simulink model "nmsRR"  (R2021a)
settings: Solver=ode15s  StartTime=0.0  StopTime=t  MaxStep=1e-2  RelTol=1e-2
StartFcn:
  | tic
StopFcn:
  | toc
  | 
  | 
  | %if GimbalLockFlag
  |  % fprintf(2, 'Almost reached Gimbal Lock of IMU. Simulation stopped.\n')
  | %end
  | 
  | %fprintf('Elapsed time: %4.2f sec (%4.2f%% realtime)\n', a, tout(end)/a*100)
undefined symbols (not defined in the file): Balance02, Balance13, BalanceTrunk, BasisStim, CompensateSwing, CompliantLeg, FlexAnkle, Ground, ICs, init_des_left, init_des_right, init_l_left, init_l_right, init_q_del, init_sensor_body, init_sensor_world, init_v_left, init_v_right, LateralControl, mParams, PreventKneeOverextension, StepDur, Target02, Target13, theta0, X, Y, Z
libraries: simulink_extras x133, nesl_utility x105, sm_lib x88, simulink x72, robotcorelib x5, dspinverses x5, dspswit3 x2, vrlib x2, robotmaniplib x1
(part 1 of 8)
settings Model: Creator=hgeyer  LastModifiedBy=reimajbi
settings SolverCC: ZeroCrossAlgorithm=Adaptive  AlgebraicLoopSolver=TrustRegion  MinimalZcImpactIntegration=on
settings OptimizationCC: EfficientMapNaN2IntZero=off
settings DebuggingCC: ReadBeforeWriteMsg=DisableAll  WriteAfterWriteMsg=DisableAll  WriteAfterReadMsg=DisableAll  IgnoredZcDiagnostic=none  MultiTaskDSMMsg=none  SFMachineParentedDataDiag=warning  ArithmeticOperatorsInVariantConditions=warning
settings HardwareCC: TargetBitPerLong=64  TargetBitPerPointer=64  TargetBitPerSizeT=64  TargetBitPerPtrDiffT=64  TargetLongLongMode=on  TargetIntDivRoundTo=Zero  TargetEndianess=LittleEndian  TargetWordSize=64  TargetHWDeviceType=MATLAB Host  ProdEqTarget=off
settings ModelReferenceCC: UpdateModelReferenceTargets=IfOutOfDate
settings SFSimCC: SFSimEcho=off  SimUseLocalCustomCode=off  CustomCodeUndefinedFunction=UseInterfaceOnly
settings CodeAppCC: MaxIdLength=128
settings SimscapeCC: SimscapeNormalizeSystem=off
settings ExplorerConfigSet: SimMechanicsOpenEditorOnUpdate=off  InternalSimMechanicsExplorerSettings="<ExplorerConfiguration><canonicalview>planar_xy</canonicalview><AnimationSetting><BasePlaybackSpeed>1.0</BasePlaybackSpeed><PlaybackSpeedFactor>1.0</PlaybackSpeedFactor></AnimationSetting><TilePanel><TileInfo><Tiles Columns=\"1\" Count=\"1\" Rows=\"1\"><Column Weight=\"1\"/><Row Weight=\"1\"/><Tile Height=\"1\" Width=\"1\" X=\"0\" Y=\"0\"/></Tiles></TileInfo><SceneInfo><SceneViewer><BGColor><R>0.60000002384185791</R><G>0.60000002384185791</G><B>0.60000002384185791</B></BGColor><Camera><DoPerspective>off</DoPerspective><Position><X>0.597774143722594631</X><Y>0.919449529340500282</Y><Z>14.1815791267909113</Z></Position><Center><X>0.597774143722594631</X><Y>0.919449529340500282</Y><Z>3.38181724401920292e-07</Z></Center><Up><X>0</X><Y>1</Y><Z>0</Z></Up><ViewLimDist>1</ViewLimDist><YLim>1.30566284997374105</YLim><XLim>1.60885047805753101</XLim></Camera></SceneViewer></SceneInfo></TilePanel><MechEditorPanel><Cameras/><GfxPanelCameraMap/><VideoCreator><PlaybackSpeedRatio>1.0</PlaybackSpeedRatio><FrameRate>30</FrameRate><VideoFormat>Motion JPEG AVI</VideoFormat><FrameSize>auto</FrameSize></VideoCreator></MechEditorPanel></ExplorerConfiguration>"

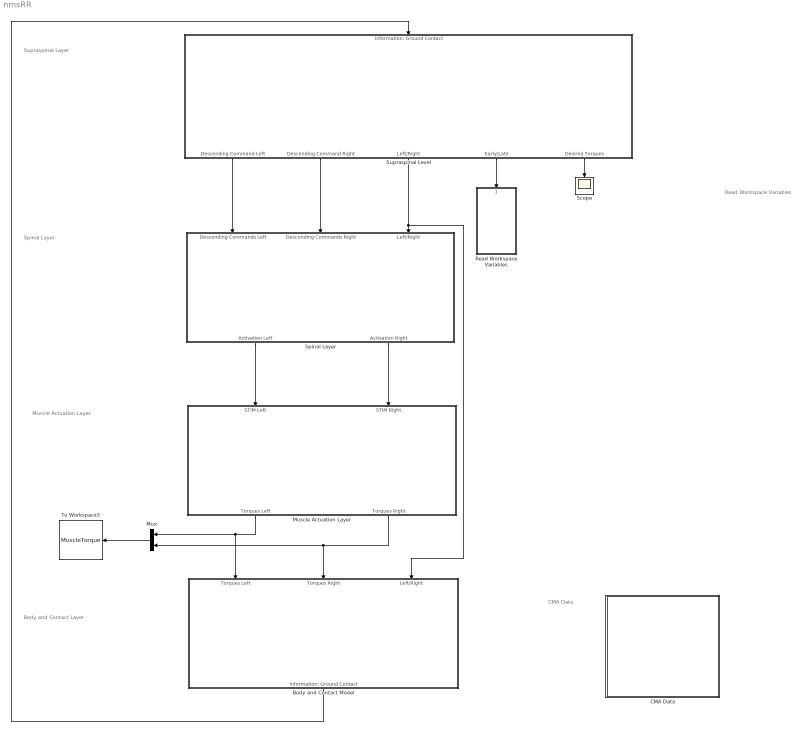
== system nmsRR ==
  note: Spinal Layer
  note: Muscle Actuation Layer
  note: Body and Contact Layer
  note: Supraspinal Layer
  note: CMA Data
  note: Read Workspace Variables
  Body and Contact Model : Subsystem
  CMA Data : Subsystem
  Muscle Actuation Layer : Subsystem
  Mux : Mux  Inputs=2
  Read Workspace Variables : Subsystem
  Scope : Scope
  Spinal Layer : Subsystem
  Supraspinal Level : Subsystem
  To Workspace3 : ToWorkspace  VariableName=MuscleTorque  SampleTime=-1
      settings: Save2DSignal=2-D array (concatenate along first dimension)
  wires:
  Spinal Layer/1(Activation Left) -> Muscle Actuation Layer/1(STIM Left)
  Spinal Layer/2(Activation Right) -> Muscle Actuation Layer/2(STIM Right)
  Muscle Actuation Layer/1(Torques Left) -> Mux/1, Body and Contact Model/1(Torques Left)
  Muscle Actuation Layer/2(Torques Right) -> Mux/2, Body and Contact Model/2(Torques Right)
  Supraspinal Level/1(Descending Command Left) -> Spinal Layer/1(Descending Commands Left)
  Supraspinal Level/2(Descending Command Right) -> Spinal Layer/2(Descending Commands Right)
  Supraspinal Level/3(Left/Right) -> Body and Contact Model/3(Left/Right), Spinal Layer/3(Left/Right)
  Supraspinal Level/4(Early/Late) -> Read Workspace Variables/1(Early/Late Swing)
  Body and Contact Model/1(Information: Ground Contact) -> Supraspinal Level/1(Information: Ground Contact)
  Mux/1 -> To Workspace3/1
  Supraspinal Level/5(Desired Torques) -> Scope/1

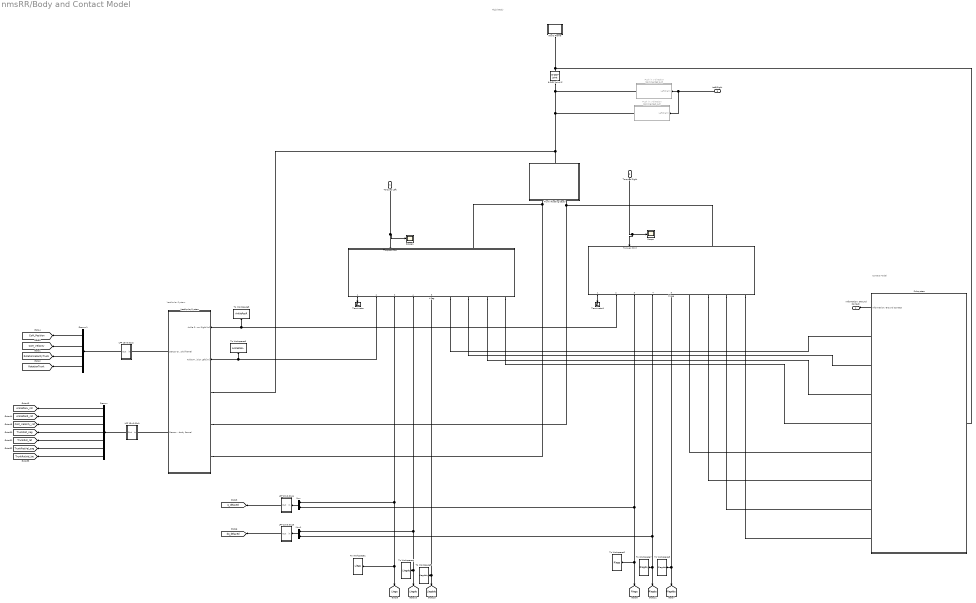
== system nmsRR/Body and Contact Model ==
  note: Rigid Body
  note: Contact Model
  note: Vestibular System
  Torques Left : Inport
  Torques Right : Inport  Port=2
  Left/Right : Inport  Port=3
  6-DOF Joint IC : sm_lib/Joints/6-DOF Joint  JointMode=Normal  SenseConstraintForce=off  SenseConstraintForceX=off  SenseConstraintForceY=off  SenseConstraintForceZ=off  SenseConstraintTorque=off  SenseConstraintTorqueX=off  SenseConstraintTorqueY=off  SenseConstraintTorqueZ=off  SenseTotalForce=off  SenseTotalForceX=off  SenseTotalForceY=off  SenseTotalForceZ=off  SenseTotalTorque=off  SenseTotalTorqueX=off  SenseTotalTorqueY=off  SenseTotalTorqueZ=off  CompositeWrenchDir=BaseOnFollower  CompositeWrenchFrame=FollowerFrame  PxEquilibriumPosition=0  PxEquilibriumPositionUnits=m  PxSpringStiffness=0  PxSpringStiffnessUnits=N/m  PxDampingCoefficient=0  PxDampingCoefficientUnits=N/(m/s)  PxTorqueActuationMode=NoTorque  PxMotionActuationMode=ComputedMotion  PxSensePosition=off  PxSenseVelocity=off  PxSenseAcceleration=off  PxSenseTorqueForce=off  PxSenseLowerLimitTorqueForce=off  PxSenseUpperLimitTorqueForce=off  PxLowerLimitSpecify=off  PxLowerLimitBound=-1  PxLowerLimitBoundUnits=m  PxLowerLimitStiffness=1e6  PxLowerLimitStiffnessUnits=N/m  PxLowerLimitDamping=1e3  PxLowerLimitDampingUnits=N/(m/s)  PxLowerLimitTransitionRegionWidth=1e-4  PxLowerLimitTransitionRegionWidthUnits=m  PxUpperLimitSpecify=off  PxUpperLimitBound=1  PxUpperLimitBoundUnits=m  PxUpperLimitStiffness=1e6  PxUpperLimitStiffnessUnits=N/m  PxUpperLimitDamping=1e3  PxUpperLimitDampingUnits=N/(m/s)  PxUpperLimitTransitionRegionWidth=1e-4  PxUpperLimitTransitionRegionWidthUnits=m  PxPositionTargetSpecify=on  PxPositionTargetPriority=High  PxPositionTargetValue=ICs.trunk.x0  PxPositionTargetValueUnits=m  PxVelocityTargetSpecify=on  PxVelocityTargetPriority=High  PxVelocityTargetValue=ICs.trunk.vx0  PxVelocityTargetValueUnits=m/s  PyEquilibriumPosition=0  PyEquilibriumPositionUnits=m  PySpringStiffness=0  PySpringStiffnessUnits=N/m  PyDampingCoefficient=0  PyDampingCoefficientUnits=N/(m/s)  PyTorqueActuationMode=NoTorque  PyMotionActuationMode=ComputedMotion  PySensePosition=off  PySenseVelocity=off  PySenseAcceleration=off  PySenseTorqueForce=off  PySenseLowerLimitTorqueForce=off  PySenseUpperLimitTorqueForce=off  PyLowerLimitSpecify=off  PyLowerLimitBound=-1  PyLowerLimitBoundUnits=m  PyLowerLimitStiffness=1e6  PyLowerLimitStiffnessUnits=N/m  PyLowerLimitDamping=1e3  PyLowerLimitDampingUnits=N/(m/s)  PyLowerLimitTransitionRegionWidth=1e-4  PyLowerLimitTransitionRegionWidthUnits=m  PyUpperLimitSpecify=off  PyUpperLimitBound=1  PyUpperLimitBoundUnits=m  PyUpperLimitStiffness=1e6  PyUpperLimitStiffnessUnits=N/m  PyUpperLimitDamping=1e3  PyUpperLimitDampingUnits=N/(m/s)  PyUpperLimitTransitionRegionWidth=1e-4  PyUpperLimitTransitionRegionWidthUnits=m  PyPositionTargetSpecify=on  PyPositionTargetPriority=High  PyPositionTargetValue=ICs.trunk.y0  PyPositionTargetValueUnits=m  PyVelocityTargetSpecify=off  PyVelocityTargetPriority=High  PyVelocityTargetValue=0  PyVelocityTargetValueUnits=m/s  PzEquilibriumPosition=0  PzEquilibriumPositionUnits=m  PzSpringStiffness=0  PzSpringStiffnessUnits=N/m  PzDampingCoefficient=0  PzDampingCoefficientUnits=N/(m/s)  PzTorqueActuationMode=NoTorque  PzMotionActuationMode=ComputedMotion  PzSensePosition=off  PzSenseVelocity=off  PzSenseAcceleration=off  PzSenseTorqueForce=off  PzSenseLowerLimitTorqueForce=off  PzSenseUpperLimitTorqueForce=off  PzLowerLimitSpecify=off  PzLowerLimitBound=-1  PzLowerLimitBoundUnits=m  PzLowerLimitStiffness=1e6  PzLowerLimitStiffnessUnits=N/m  PzLowerLimitDamping=1e3  PzLowerLimitDampingUnits=N/(m/s)  PzLowerLimitTransitionRegionWidth=1e-4  PzLowerLimitTransitionRegionWidthUnits=m  PzUpperLimitSpecify=off  PzUpperLimitBound=1  PzUpperLimitBoundUnits=m  PzUpperLimitStiffness=1e6  PzUpperLimitStiffnessUnits=N/m  PzUpperLimitDamping=1e3  PzUpperLimitDampingUnits=N/(m/s)  PzUpperLimitTransitionRegionWidth=1e-4  PzUpperLimitTransitionRegionWidthUnits=m  PzPositionTargetSpecify=on  PzPositionTargetPriority=High  PzPositionTargetValue=ICs.trunk.z0  PzPositionTargetValueUnits=m  PzVelocityTargetSpecify=on  PzVelocityTargetPriority=High  PzVelocityTargetValue=ICs.trunk.vz0  PzVelocityTargetValueUnits=m/s  SphDefPosRotationMethod=None  SphDefPosRotationAngleUnits=deg  SphDefPosRotationStandardAxis=+Z  SphDefPosRotationAngle=0.0  SphDefPosRotationArbitraryAxis=[0 0 1]  SphDefPosFollAlignAxisA=+X  SphDefPosBaseAlignAxisA=+Y  SphDefPosFollAlignAxisB=+Y  SphDefPosBaseAlignAxisB=+Z  SphDefPosRotationSequenceAxes=FollowerAxes  SphDefPosRotationSequence=XYX  SphDefPosRotationSequenceAngles=[0 0 0]  SphDefPosRotationSequenceAnglesUnits=deg  SphDefPosRotationMatrix=[1 0 0; 0 1 0; 0 0 1]  SphEqPosRotationMethod=None  SphEqPosRotationAngleUnits=deg  SphEqPosRotationStandardAxis=+Y  SphEqPosRotationAngle=0.0  SphEqPosRotationArbitraryAxis=[0 0 1]  SphEqPosFollAlignAxisA=+X  SphEqPosBaseAlignAxisA=+Y  SphEqPosFollAlignAxisB=+Y  SphEqPosBaseAlignAxisB=+Z  SphEqPosRotationSequenceAxes=FollowerAxes  SphEqPosRotationSequence=XYZ  SphEqPosRotationSequenceAngles=[0 0 -0.3]  SphEqPosRotationSequenceAnglesUnits=rad  SphEqPosRotationMatrix=[1 0 0; 0 1 0; 0 0 1]  SphSpringStiffness=0  SphSpringStiffnessUnits=N*m/deg  SphDampingCoefficient=0  SphDampingCoefficientUnits=N*m/(deg/s)  SphActuateTorqueX=off  SphActuateTorqueY=off  SphActuateTorqueZ=off  SphActuateTorque=on  SphTorqueActuationMode=NoTorque  SphMotionActuationMode=ComputedMotion  SphActuationFrame=BaseFrame  SphSensePosition=off  SphSenseVelocityX=off  SphSenseVelocityY=off  SphSenseVelocityZ=off  SphSenseVelocity=off  SphSenseAccelerationX=off  SphSenseAccelerationY=off  SphSenseAccelerationZ=off  SphSenseAcceleration=off  SphSenseTorqueX=off  SphSenseTorqueY=off  SphSenseTorqueZ=off  SphSenseTorqueForce=off  SphSenseLowerLimitTorqueMag=off  SphSenseUpperLimitTorqueMag=off  SphSensingFrame=BaseFrame  SphLowerLimitSpecify=off  SphLowerLimitBound=15  SphLowerLimitBoundUnits=deg  SphLowerLimitStiffness=1e4  SphLowerLimitStiffnessUnits=N*m/deg  SphLowerLimitDamping=10  SphLowerLimitDampingUnits=N*m/(deg/s)  SphLowerLimitTransitionRegionWidth=0.1  SphLowerLimitTransitionRegionWidthUnits=deg  SphUpperLimitSpecify=off  SphUpperLimitBound=45  SphUpperLimitBoundUnits=deg  SphUpperLimitStiffness=1e4  SphUpperLimitStiffnessUnits=N*m/deg  SphUpperLimitDamping=10  SphUpperLimitDampingUnits=N*m/(deg/s)  SphUpperLimitTransitionRegionWidth=0.1  SphUpperLimitTransitionRegionWidthUnits=deg  SphPositionTargetRotationMethod=RotationSequence  SphPositionTargetRotationAngleUnits=deg  SphPositionTargetRotationStandardAxis=+Z  SphPositionTargetRotationAngle=0.0  SphPositionTargetRotationArbitraryAxis=[0 0 1]  SphPositionTargetFollAlignAxisA=+X  SphPositionTargetBaseAlignAxisA=+Y  SphPositionTargetFollAlignAxisB=+Y  SphPositionTargetBaseAlignAxisB=+Z  SphPositionTargetRotationSequenceAxes=BaseAxes  SphPositionTargetRotationSequence=XZY  SphPositionTargetRotationSequenceAngles=[ICs.trunk.qR0 ICs.trunk.qP0 ICs.trunk.qY0 ]  SphPositionTargetRotationSequenceAnglesUnits=rad  SphPositionTargetRotationMatrix=[1 0 0; 0 1 0; 0 0 1]  SphPositionTargetSpecify=on  SphPositionTargetPriority=High  SphVelocityTargetValue=[ICs.trunk.qR0 ICs.trunk.qP0 ICs.trunk.qY0 ]  SphVelocityTargetValueUnits=deg/s  SphVelocityTargetSpecify=on  SphVelocityTargetPriority=High  SphVelocityTargetInFollowerFrame=on
  Demux : Demux  Outputs=7
  Demux1 : Demux
  L Leg : Subsystem
  LPF 13x0.01s1 : Subsystem
  LPF 13x0.01s2 : Subsystem
  LPF 13x0.01s3 : Subsystem
  LPF 13x0.01s4 : Subsystem
  Mux : Mux  Inputs=2
  Mux1 : Mux  Inputs=2
  Push in x-direction : Subsystem  Commented=on
  Push in y-direction : Subsystem  Commented=on
  R Leg : Subsystem
  Scope : Scope
  Scope1 : Scope
  Subsystem : Subsystem
  Terminator : Terminator
  Terminator1 : Terminator
  To Workspace1 : ToWorkspace  VariableName=Llegq  SampleTime=-1
      settings: Save2DSignal=2-D array (concatenate along first dimension)
  To Workspace2 : ToWorkspace  VariableName=Rlegq  SampleTime=-1
      settings: Save2DSignal=2-D array (concatenate along first dimension)
  To Workspace3 : ToWorkspace  VariableName=AnklePosR  SampleTime=-1
      settings: Save2DSignal=2-D array (concatenate along first dimension)
  To Workspace4 : ToWorkspace  VariableName=Llegdq  SampleTime=-1
      settings: Save2DSignal=2-D array (concatenate along first dimension)
  To Workspace5 : ToWorkspace  VariableName=Llegddq  SampleTime=-1
      settings: Save2DSignal=2-D array (concatenate along first dimension)
  To Workspace6 : ToWorkspace  VariableName=AnklePosL  SampleTime=-1
      settings: Save2DSignal=2-D array (concatenate along first dimension)
  To Workspace7 : ToWorkspace  VariableName=Rlegdq  SampleTime=-1
      settings: Save2DSignal=2-D array (concatenate along first dimension)
  To Workspace8 : ToWorkspace  VariableName=Rlegddq  SampleTime=-1
      settings: Save2DSignal=2-D array (concatenate along first dimension)
  Trunk (floating base) : Subsystem
  Vestibular System : Subsystem
  World Frame : Subsystem
  Information: Ground Contact : Outport
  tag scope: AnklePosL_rot=global, AnklePosR_rot=global, CoM_Position=global, CoM_Velocity=global, CoM_Velocity_rot=global, Llegddq=global, Llegdq=global, Llegq=global, Rlegddq=global, Rlegdq=global, Rlegq=global, RotationTrunk=global, RotationVelocityTrunk=global, TrunkRotVel_lat=global, TrunkRotVel_sag=global, TrunkRot_lat=global, TrunkRot_sag=global, dq_delayed=global, q_delayed=global
  wires:
  R Leg/4("Joint Velocities Right [rad/s] ") -> Mux1/2, To Workspace7/1, [Rlegdq]
  R Leg/5(Joint Accelerations Right [rad/s^2]) -> To Workspace8/1, [Rlegddq]
  R Leg/3(Joint Angles Right [rad]) -> Mux/2, To Workspace2/1, [Rlegq]
  L Leg/3(Joint Angles Left [rad]) -> Mux/1, To Workspace1/1, [Llegq]
  L Leg/5(Joint Accelerations Left [rad/s^2]) -> To Workspace5/1, [Llegddq]
  L Leg/4("Joint Velocities Left [rad/s] ") -> To Workspace4/1, [Llegdq], Mux1/1
  R Leg/2(Position Right Ankle [m]) -> To Workspace3/1, Vestibular System/1(Ankle Position Right [m])
  L Leg/2(" Position Left Ankle [m]") -> To Workspace6/1, Vestibular System/2(Ankle Position Left [m])
  Subsystem/1(Information: Ground Contact) -> Information: Ground Contact/1
  Demux1/2 -> [CoM_Velocity]
  Demux/3 -> [CoM_Velocity_rot]
  Vestibular System/2(Sensor Data (body frame)) -> LPF 13x0.01s1/1(in)
  Demux/5 -> [TrunkRot_lat]
  Demux/6 -> [TrunkRotVel_sag]
  Demux1/1 -> [CoM_Position]
  Demux/4 -> [TrunkRot_sag]
  Demux1/4 -> [RotationTrunk]
  Demux/2 -> [AnklePosR_rot]
  Demux1/3 -> [RotationVelocityTrunk]
  Demux/1 -> [AnklePosL_rot]
  Demux/7 -> [TrunkRotVel_lat]
  L Leg/1(Rotation Matrix Left Knee (world)) -> Terminator/1
  R Leg/1(Rotation Matrix Right Knee (World)) -> Terminator1/1
  Left/Right/1 -> Push in y-direction/1(Left/Right), Push in x-direction/1(Left/Right)
  Mux/1 -> LPF 13x0.01s4/1(in)
  Mux1/1 -> LPF 13x0.01s3/1(in)
  Torques Left/1 -> Scope1/1, L Leg/1(Torques [Nm])
  Torques Right/1 -> Scope/1, R Leg/1(Torques [Nm])
  LPF 13x0.01s2/1(Out) -> Demux1/1
  LPF 13x0.01s1/1(Out) -> Demux/1
  Vestibular System/1(Sensor Data (world frame)) -> LPF 13x0.01s2/1(in)
  LPF 13x0.01s4/1(Out) -> [q_delayed]
  LPF 13x0.01s3/1(Out) -> [dq_delayed]
  connections:
  Trunk (floating base)/RConn1 -- Vestibular System/LConn3 -- L Leg/LConn1
  World Frame/RConn1 -- Subsystem/LConn1 -- 6-DOF Joint IC/LConn1
  L Leg/RConn1 -- Subsystem/RConn1
  L Leg/RConn2 -- Subsystem/RConn2
  L Leg/RConn3 -- Subsystem/RConn3
  L Leg/RConn4 -- Subsystem/RConn4
  Subsystem/RConn5 -- R Leg/RConn1
  R Leg/RConn2 -- Subsystem/RConn6
  R Leg/RConn3 -- Subsystem/RConn7
  R Leg/RConn4 -- Subsystem/RConn8
  Vestibular System/LConn2 -- R Leg/LConn1 -- Trunk (floating base)/RConn2
  6-DOF Joint IC/RConn1 -- Push in x-direction/RConn1 -- Push in y-direction/RConn1 -- Vestibular System/LConn1 -- Trunk (floating base)/LConn1

== system nmsRR/CMA Data ==
  Mux : Mux  Inputs=7
  SS_dist1 : Subsystem  TreatAsAtomicUnit=on
  Step Counter : Subsystem
  check steady state : Subsystem
  wires:
  Step Counter/1(nStep) -> check steady state/2(nStep)
  [Contact_left] -> Step Counter/2(Step1), SS_dist1/Trigger
  [Contact_right] -> Step Counter/1(Step2)
  [Ball_right] -> Mux/1
  [AnklePosR] -> Mux/2
  [HipR] -> Mux/3
  [TRK_CG] -> Mux/4
  [HipL] -> Mux/5
  [Ball_left] -> Mux/6
  [AnklePosL] -> Mux/7
  Mux/1 -> check steady state/1(p)
  check steady state/1(SS_dist) -> SS_dist1/1(In1)

== system nmsRR/Muscle Actuation Layer ==
  note: Muscle Actuation Layer
  STIM Left : Inport
  STIM Right : Inport  Port=2
  Muscles Left : Subsystem
  Muscles Right : Subsystem
  Mux : Mux
  Mux1 : Mux
  Torques Left : Outport
  Torques Right : Outport  Port=2
  wires:
  STIM Left/1 -> Muscles Left/1(STIM Left)
  STIM Right/1 -> Muscles Right/1(STIM Right)
  Muscles Left/1(tauHipPitchL) -> Mux/1
  Muscles Left/2(tauHipRollL) -> Mux/2
  Muscles Left/3(tauKneeL) -> Mux/3
  Muscles Left/4(tauHipAnkleL) -> Mux/4
  Muscles Right/1(tauHipPitchR) -> Mux1/1
  Muscles Right/2(tauHipRollR) -> Mux1/2
  Muscles Right/3(tauKneeR) -> Mux1/3
  Muscles Right/4(tauHipAnkleR) -> Mux1/4
  Mux/1 -> Torques Left/1
  Mux1/1 -> Torques Right/1

== system nmsRR/Read Workspace Variables ==
  Early/Late Swing : Inport
  Constant : Constant  Value=0
  Constant1 : Constant  Value=CompliantLeg
  Constant10 : Constant  Value=theta0
  Constant12 : Constant  Value=BasisStim
  Constant15 : Constant  Value=LateralControl
  Constant2 : Constant  Value=CompensateSwing
  Constant3 : Constant  Value=Balance02
  Constant4 : Constant  Value=Target02
  Constant5 : Constant  Value=Balance13
  Constant6 : Constant  Value=Target13
  Constant7 : Constant  Value=PreventKneeOverextension
  Constant8 : Constant  Value=BalanceTrunk
  Constant9 : Constant  Value=FlexAnkle
  Demux : Demux
  Demux1 : Demux  Outputs=2
  Mux : Mux  Inputs=5
  Switch1 : Switch  Criteria=u2 > Threshold
  Switch2 : Switch  Criteria=u2 > Threshold
  tag scope: BasisStim=global, ControlParam=global, ControlParamLat=global, cd=global, cd_lat=global, cv=global, cv_lat=global, swh=global, swh_lat=global, swk=global, theta0=global
  wires:
  Constant2/1 -> Mux/5
  Constant5/1 -> Switch2/3
  Constant1/1 -> Mux/1
  Demux/2 -> [cv]
  Switch2/1 -> Demux/1
  Constant3/1 -> Switch2/1
  Mux/1 -> [ControlParam]
  Constant8/1 -> Mux/3
  Demux/3 -> [cd_lat]
  Constant9/1 -> Mux/4
  Constant15/1 -> [ControlParamLat]
  Demux/1 -> [cd]
  Constant12/1 -> [BasisStim]
  Constant7/1 -> Mux/2
  Demux/4 -> [cv_lat]
  Constant/1 -> [swh_lat]
  Early/Late Swing/1 -> Switch1/2, Switch2/2
  Constant6/1 -> Switch1/3
  Switch1/1 -> Demux1/1
  Constant4/1 -> Switch1/1
  Demux1/1 -> [swh]
  Demux1/2 -> [swk]
  Constant10/1 -> [theta0]

== system nmsRR/Spinal Layer ==
  Descending Commands Left : Inport
  Descending Commands Right : Inport  Port=2
  Left/Right : Inport  Port=3
  Stance Leg Control Left : Subsystem
  Stance Leg Control Right : Subsystem
  Stretch Reflex for Swing Leg Control : Subsystem
  Switch : Switch  Criteria=u2 > Threshold
  Switch1 : Switch  Criteria=u2 > Threshold
  Activation Left : Outport
  Activation Right : Outport  Port=2
  wires:
  Descending Commands Right/1 -> Stretch Reflex for Swing Leg Control/2(Descending Commands Right)
  Descending Commands Left/1 -> Stretch Reflex for Swing Leg Control/1(Descending Commands Left)
  Stance Leg Control Right/1(Activation Right) -> Switch/3
  Left/Right/1 -> Switch1/2, Switch/2
  Stretch Reflex for Swing Leg Control/1(Activation Left) -> Stance Leg Control Right/1(Activation Swing Left), Switch1/3
  Stance Leg Control Left/1(Activation Left) -> Switch1/1
  Stretch Reflex for Swing Leg Control/2(Activation Right) -> Stance Leg Control Left/1(Activation Swing Right), Switch/1
  Switch1/1 -> Activation Left/1
  Switch/1 -> Activation Right/1

== system nmsRR/Supraspinal Level ==
  note: Finite State Machine
  note: Descending Commands for Swing Leg Control
  note: input: ground contact
  note: output: descending commands
  Information: Ground Contact : Inport
  Early/ Late : Logic  Operator=OR  AllPortsSameDT=off  OutDataTypeStr=boolean
  Finite State Machine : Subsystem
  Left/ Right : Logic  Operator=OR  AllPortsSameDT=off  OutDataTypeStr=boolean
  Subsystem : Subsystem
  To Workspace1 : ToWorkspace  VariableName=LateRight  SampleTime=-1
      settings: Save2DSignal=2-D array (concatenate along first dimension)
  To Workspace2 : ToWorkspace  VariableName=EarlyRight  SampleTime=-1
      settings: Save2DSignal=2-D array (concatenate along first dimension)
  To Workspace3 : ToWorkspace  VariableName=EarlyLeft  SampleTime=-1
      settings: Save2DSignal=2-D array (concatenate along first dimension)
  To Workspace4 : ToWorkspace  VariableName=Contact  SampleTime=-1
      settings: Save2DSignal=2-D array (concatenate along first dimension)
  To Workspace5 : ToWorkspace  VariableName=LateLeft  SampleTime=-1
      settings: Save2DSignal=2-D array (concatenate along first dimension)
  Descending Command Left : Outport
  Descending Command Right : Outport  Port=2
  Left/Right : Outport  Port=3
  Early/Late : Outport  Port=4
  Desired Torques : Outport  Port=5
  wires:
  Finite State Machine/3(Early Left Swing) -> Early/ Late/2, To Workspace3/1
  Left/ Right/1 -> Left/Right/1, Subsystem/2(Left/Right)
  Finite State Machine/1(Early Right Swing) -> To Workspace2/1, Left/ Right/1, Early/ Late/1
  Finite State Machine/4(Late Left Swing) -> To Workspace5/1
  Finite State Machine/2(Late Right Swing) -> Left/ Right/2, To Workspace1/1
  Early/ Late/1 -> Early/Late/1, Subsystem/1(Early/Late Swing)
  Information: Ground Contact/1 -> Finite State Machine/1(Information: Ground Contact), To Workspace4/1
  Subsystem/1(Descending Command Left) -> Descending Command Left/1
  Subsystem/2(Descending Command Right) -> Descending Command Right/1
  Subsystem/3(Desired Torques) -> Desired Torques/1

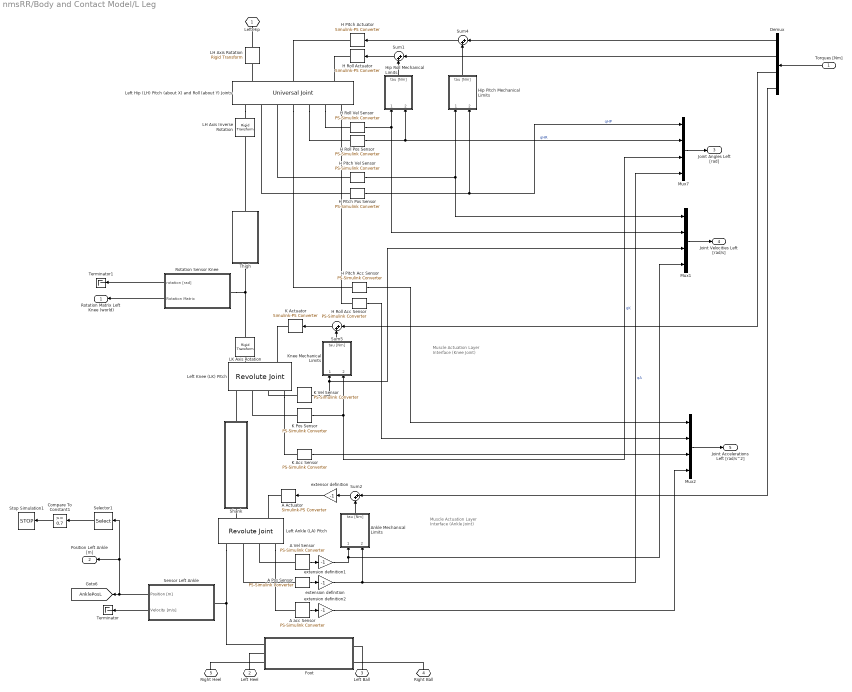
== system nmsRR/Body and Contact Model/L Leg ==
  note: Muscle Actuation
      | Layer Interface
      | (Ankle Joint)
  note: Muscle Actuation
      | Layer Interface
      | (Knee Joint)
  Torques [Nm] : Inport
  " K Actuator" : nesl_utility/Simulink-PS Converter  PhysicalDomain=network_engine_domain  SubClassName=ps_input  LeftPortType=input  RightPortType=output  PseudoPeriodic=off  Frequencies=[]  NoiseDistribution=none  NoiseParameters=[]  Unit=N*m  AffineConversion=off  FilteringAndDerivatives=zero  SimscapeFilterOrder=1  InputFilterTimeConstant=.001  UdotUserProvided=0
      settings: SourceProductBaseCode=PW,SS
  A Actuator : nesl_utility/Simulink-PS Converter  PhysicalDomain=network_engine_domain  SubClassName=ps_input  LeftPortType=input  RightPortType=output  PseudoPeriodic=off  Frequencies=[]  NoiseDistribution=none  NoiseParameters=[]  Unit=N*m  AffineConversion=off  FilteringAndDerivatives=zero  SimscapeFilterOrder=1  InputFilterTimeConstant=.001  UdotUserProvided=0
      settings: SourceProductBaseCode=PW,SS
  A Pos Sensor : nesl_utility/PS-Simulink Converter  PhysicalDomain=network_engine_domain  SubClassName=ps_output  LeftPortType=input  RightPortType=output  PseudoPeriodic=off  Frequencies=[]  Unit=rad  AffineConversion=off
      settings: SourceProductBaseCode=PW,SS
  A Vel Sensor : nesl_utility/PS-Simulink Converter  PhysicalDomain=network_engine_domain  SubClassName=ps_output  LeftPortType=input  RightPortType=output  PseudoPeriodic=off  Frequencies=[]  Unit=rad/s  AffineConversion=off
      settings: SourceProductBaseCode=PW,SS
  A acc Sensor : nesl_utility/PS-Simulink Converter  PhysicalDomain=network_engine_domain  SubClassName=ps_output  LeftPortType=input  RightPortType=output  PseudoPeriodic=off  Frequencies=[]  Unit=rad/(s^2)  AffineConversion=off
      settings: SourceProductBaseCode=PW,SS
  Ankle Mechanical Limits : Subsystem
  Compare To Constant1 : simulink/Logic and Bit Operations/Compare To Constant  relop=>=  const=0.7  OutDataTypeStr=boolean
  Demux : Demux
  Foot : Subsystem
  H Pitch Actuator : nesl_utility/Simulink-PS Converter  PhysicalDomain=network_engine_domain  SubClassName=ps_input  LeftPortType=input  RightPortType=output  PseudoPeriodic=off  Frequencies=[]  NoiseDistribution=none  NoiseParameters=[]  Unit=N*m  AffineConversion=off  FilteringAndDerivatives=zero  SimscapeFilterOrder=1  InputFilterTimeConstant=.001  UdotUserProvided=0
      settings: SourceProductBaseCode=PW,SS
  H Pitch Acc Sensor : nesl_utility/PS-Simulink Converter  PhysicalDomain=network_engine_domain  SubClassName=ps_output  LeftPortType=input  RightPortType=output  PseudoPeriodic=off  Frequencies=[]  Unit=rad/(s^2)  AffineConversion=off
      settings: SourceProductBaseCode=PW,SS
  H Pitch Pos Sensor : nesl_utility/PS-Simulink Converter  PhysicalDomain=network_engine_domain  SubClassName=ps_output  LeftPortType=input  RightPortType=output  PseudoPeriodic=off  Frequencies=[]  Unit=rad  AffineConversion=off
      settings: SourceProductBaseCode=PW,SS
  H Pitch Vel Sensor : nesl_utility/PS-Simulink Converter  PhysicalDomain=network_engine_domain  SubClassName=ps_output  LeftPortType=input  RightPortType=output  PseudoPeriodic=off  Frequencies=[]  Unit=rad/s  AffineConversion=off
      settings: SourceProductBaseCode=PW,SS
  H Roll Actuator : nesl_utility/Simulink-PS Converter  PhysicalDomain=network_engine_domain  SubClassName=ps_input  LeftPortType=input  RightPortType=output  PseudoPeriodic=off  Frequencies=[]  NoiseDistribution=none  NoiseParameters=[]  Unit=N*m  AffineConversion=off  FilteringAndDerivatives=zero  SimscapeFilterOrder=1  InputFilterTimeConstant=.001  UdotUserProvided=0
      settings: SourceProductBaseCode=PW,SS
  H Roll Acc Sensor : nesl_utility/PS-Simulink Converter  PhysicalDomain=network_engine_domain  SubClassName=ps_output  LeftPortType=input  RightPortType=output  PseudoPeriodic=off  Frequencies=[]  Unit=rad/(s^2)  AffineConversion=off
      settings: SourceProductBaseCode=PW,SS
  H Roll Pos Sensor : nesl_utility/PS-Simulink Converter  PhysicalDomain=network_engine_domain  SubClassName=ps_output  LeftPortType=input  RightPortType=output  PseudoPeriodic=off  Frequencies=[]  Unit=rad  AffineConversion=off
      settings: SourceProductBaseCode=PW,SS
  "H Roll Vel Sensor " : nesl_utility/PS-Simulink Converter  PhysicalDomain=network_engine_domain  SubClassName=ps_output  LeftPortType=input  RightPortType=output  PseudoPeriodic=off  Frequencies=[]  Unit=rad/s  AffineConversion=off
      settings: SourceProductBaseCode=PW,SS
  Hip Pitch Mechanical Limits : Subsystem
  Hip Roll Mechanical Limits : Subsystem
  K Acc Sensor : nesl_utility/PS-Simulink Converter  PhysicalDomain=network_engine_domain  SubClassName=ps_output  LeftPortType=input  RightPortType=output  PseudoPeriodic=off  Frequencies=[]  Unit=rad/(s^2)  AffineConversion=off
      settings: SourceProductBaseCode=PW,SS
  K Pos Sensor : nesl_utility/PS-Simulink Converter  PhysicalDomain=network_engine_domain  SubClassName=ps_output  LeftPortType=input  RightPortType=output  PseudoPeriodic=off  Frequencies=[]  Unit=rad  AffineConversion=off
      settings: SourceProductBaseCode=PW,SS
  K Vel Sensor : nesl_utility/PS-Simulink Converter  PhysicalDomain=network_engine_domain  SubClassName=ps_output  LeftPortType=input  RightPortType=output  PseudoPeriodic=off  Frequencies=[]  Unit=rad/s  AffineConversion=off
      settings: SourceProductBaseCode=PW,SS
  Knee Mechanical Limits : Subsystem
  LH Axis Inverse Rotation : sm_lib/Frames and Transforms/Rigid Transform  TranslationMethod=None  TranslationStandardOffset=-0.2  TranslationLengthUnit=m  TranslationStandardAxis=+Y  TranslationCartesianOffset=0  TranslationROffset=0  TranslationROffsetUnits=m  TranslationZOffset=0  TranslationZOffsetUnits=m  TranslationThetaOffset=0  TranslationThetaOffsetUnits=deg  RotationMethod=RotationSequence  RotationAngleUnits=deg  RotationStandardAxis=+X  RotationAngle=-90  RotationArbitraryAxis=[0 0 1]  FollAlignAxisA=+X  BaseAlignAxisA=+Y  FollAlignAxisB=+Y  BaseAlignAxisB=+Z  RotationSequenceAxes=BaseAxes  RotationSequence=YXY  RotationSequenceAngles=[-90 -90 0]  RotationSequenceAnglesUnits=deg  RotationMatrix=[1 0 0; 0 1 0; 0 0 1]
  LH Axis Rotation : sm_lib/Frames and Transforms/Rigid Transform  TranslationMethod=None  TranslationStandardOffset=-0.2  TranslationLengthUnit=m  TranslationStandardAxis=+Y  TranslationCartesianOffset=0  TranslationROffset=0  TranslationROffsetUnits=m  TranslationZOffset=0  TranslationZOffsetUnits=m  TranslationThetaOffset=0  TranslationThetaOffsetUnits=deg  RotationMethod=RotationSequence  RotationAngleUnits=deg  RotationStandardAxis=+X  RotationAngle=90  RotationArbitraryAxis=[0 0 1]  FollAlignAxisA=+X  BaseAlignAxisA=+Y  FollAlignAxisB=+Y  BaseAlignAxisB=+Z  RotationSequenceAxes=FollowerAxes  RotationSequence=XZX  RotationSequenceAngles=[-90 90 0]  RotationSequenceAnglesUnits=deg  RotationMatrix=[1 0 0; 0 1 0; 0 0 1]
  LK Axis Rotation : sm_lib/Frames and Transforms/Rigid Transform  TranslationMethod=None  TranslationStandardOffset=-0.5  TranslationLengthUnit=m  TranslationStandardAxis=+Y  TranslationCartesianOffset=0  TranslationROffset=0  TranslationROffsetUnits=m  TranslationZOffset=0  TranslationZOffsetUnits=m  TranslationThetaOffset=0  TranslationThetaOffsetUnits=deg  RotationMethod=RotationSequence  RotationAngleUnits=deg  RotationStandardAxis=+X  RotationAngle=-90  RotationArbitraryAxis=[0 0 1]  FollAlignAxisA=+X  BaseAlignAxisA=+Y  FollAlignAxisB=+Y  BaseAlignAxisB=+Z  RotationSequenceAxes=BaseAxes  RotationSequence=ZXZ  RotationSequenceAngles=[180 0 0]  RotationSequenceAnglesUnits=deg  RotationMatrix=[1 0 0; 0 1 0; 0 0 1]
  Left Ankle (LA) Pitch : sm_lib/Joints/Revolute Joint  JointMode=Normal  SenseConstraintForce=off  SenseConstraintForceX=off  SenseConstraintForceY=off  SenseConstraintForceZ=off  SenseConstraintTorque=off  SenseConstraintTorqueX=off  SenseConstraintTorqueY=off  SenseConstraintTorqueZ=off  SenseTotalForce=off  SenseTotalForceX=off  SenseTotalForceY=off  SenseTotalForceZ=off  SenseTotalTorque=off  SenseTotalTorqueX=off  SenseTotalTorqueY=off  SenseTotalTorqueZ=off  CompositeWrenchDir=FollowerOnBase  CompositeWrenchFrame=FollowerFrame  EquilibriumPosition=0  EquilibriumPositionUnits=deg  SpringStiffness=0  SpringStiffnessUnits=N*m/deg  DampingCoefficient=0  DampingCoefficientUnits=N*m/(deg/s)  TorqueActuationMode=InputTorque  MotionActuationMode=ComputedMotion  SensePosition=on  SenseVelocity=on  SenseAcceleration=on  SenseTorqueForce=off  SenseLowerLimitTorqueForce=off  SenseUpperLimitTorqueForce=off  LowerLimitSpecify=off  LowerLimitBound=-90  LowerLimitBoundUnits=deg  LowerLimitStiffness=1e4  LowerLimitStiffnessUnits=N*m/deg  LowerLimitDamping=10  LowerLimitDampingUnits=N*m/(deg/s)  LowerLimitTransitionRegionWidth=0.1  LowerLimitTransitionRegionWidthUnits=deg  UpperLimitSpecify=off  UpperLimitBound=90  UpperLimitBoundUnits=deg  UpperLimitStiffness=1e4  UpperLimitStiffnessUnits=N*m/deg  UpperLimitDamping=10  UpperLimitDampingUnits=N*m/(deg/s)  UpperLimitTransitionRegionWidth=0.1  UpperLimitTransitionRegionWidthUnits=deg  PositionTargetSpecify=on  PositionTargetPriority=High  PositionTargetValue=-ICs.lLeg.ankle.qP0  PositionTargetValueUnits=rad  VelocityTargetSpecify=on  VelocityTargetPriority=High  VelocityTargetValue=0  VelocityTargetValueUnits=rad/s
  Left Hip (LH) Pitch (about X) and Roll (about Y) Joints : sm_lib/Joints/Universal Joint  JointMode=Normal  SenseConstraintForce=off  SenseConstraintForceX=off  SenseConstraintForceY=off  SenseConstraintForceZ=off  SenseConstraintTorque=off  SenseConstraintTorqueX=off  SenseConstraintTorqueY=off  SenseConstraintTorqueZ=off  SenseTotalForce=off  SenseTotalForceX=off  SenseTotalForceY=off  SenseTotalForceZ=off  SenseTotalTorque=off  SenseTotalTorqueX=off  SenseTotalTorqueY=off  SenseTotalTorqueZ=off  CompositeWrenchDir=FollowerOnBase  CompositeWrenchFrame=FollowerFrame  RxEquilibriumPosition=0  RxEquilibriumPositionUnits=deg  RxSpringStiffness=0  RxSpringStiffnessUnits=N*m/deg  RxDampingCoefficient=0  RxDampingCoefficientUnits=N*m/(deg/s)  RxTorqueActuationMode=InputTorque  RxMotionActuationMode=ComputedMotion  RxSensePosition=on  RxSenseVelocity=on  RxSenseAcceleration=on  RxSenseTorqueForce=off  RxSenseLowerLimitTorqueForce=off  RxSenseUpperLimitTorqueForce=off  RxLowerLimitSpecify=off  RxLowerLimitBound=-90  RxLowerLimitBoundUnits=deg  RxLowerLimitStiffness=1e4  RxLowerLimitStiffnessUnits=N*m/deg  RxLowerLimitDamping=10  RxLowerLimitDampingUnits=N*m/(deg/s)  RxLowerLimitTransitionRegionWidth=0.1  RxLowerLimitTransitionRegionWidthUnits=deg  RxUpperLimitSpecify=off  RxUpperLimitBound=90  RxUpperLimitBoundUnits=deg  RxUpperLimitStiffness=1e4  RxUpperLimitStiffnessUnits=N*m/deg  RxUpperLimitDamping=10  RxUpperLimitDampingUnits=N*m/(deg/s)  RxUpperLimitTransitionRegionWidth=0.1  RxUpperLimitTransitionRegionWidthUnits=deg  RxPositionTargetSpecify=on  RxPositionTargetPriority=High  RxPositionTargetValue=ICs.lLeg.hip.qP0  RxPositionTargetValueUnits=rad  RxVelocityTargetSpecify=on  RxVelocityTargetPriority=High  RxVelocityTargetValue=0  RxVelocityTargetValueUnits=rad/s  RyEquilibriumPosition=0  RyEquilibriumPositionUnits=deg  RySpringStiffness=0  RySpringStiffnessUnits=N*m/deg  RyDampingCoefficient=0  RyDampingCoefficientUnits=N*m/(deg/s)  RyTorqueActuationMode=InputTorque  RyMotionActuationMode=ComputedMotion  RySensePosition=on  RySenseVelocity=on  RySenseAcceleration=on  RySenseTorqueForce=off  RySenseLowerLimitTorqueForce=off  RySenseUpperLimitTorqueForce=off  RyLowerLimitSpecify=off  RyLowerLimitBound=-90  RyLowerLimitBoundUnits=deg  RyLowerLimitStiffness=1e4  RyLowerLimitStiffnessUnits=N*m/deg  RyLowerLimitDamping=10  RyLowerLimitDampingUnits=N*m/(deg/s)  RyLowerLimitTransitionRegionWidth=0.1  RyLowerLimitTransitionRegionWidthUnits=deg  RyUpperLimitSpecify=off  RyUpperLimitBound=90  RyUpperLimitBoundUnits=deg  RyUpperLimitStiffness=1e4  RyUpperLimitStiffnessUnits=N*m/deg  RyUpperLimitDamping=10  RyUpperLimitDampingUnits=N*m/(deg/s)  RyUpperLimitTransitionRegionWidth=0.1  RyUpperLimitTransitionRegionWidthUnits=deg  RyPositionTargetSpecify=on  RyPositionTargetPriority=High  RyPositionTargetValue=ICs.lLeg.hip.qR0  RyPositionTargetValueUnits=rad  RyVelocityTargetSpecify=on  RyVelocityTargetPriority=High  RyVelocityTargetValue=0  RyVelocityTargetValueUnits=rad/s
  Left Knee (LK) Pitch : sm_lib/Joints/Revolute Joint  JointMode=Normal  SenseConstraintForce=off  SenseConstraintForceX=off  SenseConstraintForceY=off  SenseConstraintForceZ=off  SenseConstraintTorque=off  SenseConstraintTorqueX=off  SenseConstraintTorqueY=off  SenseConstraintTorqueZ=off  SenseTotalForce=off  SenseTotalForceX=off  SenseTotalForceY=off  SenseTotalForceZ=off  SenseTotalTorque=off  SenseTotalTorqueX=off  SenseTotalTorqueY=off  SenseTotalTorqueZ=off  CompositeWrenchDir=FollowerOnBase  CompositeWrenchFrame=FollowerFrame  EquilibriumPosition=0  EquilibriumPositionUnits=deg  SpringStiffness=0  SpringStiffnessUnits=N*m/deg  DampingCoefficient=0  DampingCoefficientUnits=N*m/(deg/s)  TorqueActuationMode=InputTorque  MotionActuationMode=ComputedMotion  SensePosition=on  SenseVelocity=on  SenseAcceleration=on  SenseTorqueForce=off  SenseLowerLimitTorqueForce=off  SenseUpperLimitTorqueForce=off  LowerLimitSpecify=off  LowerLimitBound=-90  LowerLimitBoundUnits=deg  LowerLimitStiffness=1e4  LowerLimitStiffnessUnits=N*m/deg  LowerLimitDamping=10  LowerLimitDampingUnits=N*m/(deg/s)  LowerLimitTransitionRegionWidth=0.1  LowerLimitTransitionRegionWidthUnits=deg  UpperLimitSpecify=off  UpperLimitBound=90  UpperLimitBoundUnits=deg  UpperLimitStiffness=1e4  UpperLimitStiffnessUnits=N*m/deg  UpperLimitDamping=10  UpperLimitDampingUnits=N*m/(deg/s)  UpperLimitTransitionRegionWidth=0.1  UpperLimitTransitionRegionWidthUnits=deg  PositionTargetSpecify=on  PositionTargetPriority=High  PositionTargetValue=ICs.lLeg.knee.qP0  PositionTargetValueUnits=rad  VelocityTargetSpecify=on  VelocityTargetPriority=High  VelocityTargetValue=0  VelocityTargetValueUnits=rad/s
  Mux1 : Mux
  Mux2 : Mux
  Mux7 : Mux
  Rotation Sensor Knee : Subsystem
  Selector1 : Selector  InputPortWidth=3  IndexOptions=Index vector (dialog)  Indices=[2]  OutputSizes=1
  Sensor Left Ankle : Subsystem
  Shank : Subsystem
  Stop Simulation1 : Stop
  Sum{1..2,4..5} (4 alike) : Sum  Inputs=|++
  Terminator : Terminator
  Terminator1 : Terminator
  Thigh : Subsystem
  extension definition : Gain  Gain=-1
  extension definition1 : Gain  Gain=-1
  extension definition2 : Gain  Gain=-1
  extensor definition : Gain  Gain=-1
  Left Hip : PMIOPort  Side=Left
  Left Heel : PMIOPort  Port=2  Side=Right
  Left Ball : PMIOPort  Port=3  Side=Right
  Right Ball : PMIOPort  Port=4  Side=Right
  Right Heel : PMIOPort  Port=5  Side=Right
  Rotation Matrix Left Knee (world) : Outport
  " Position Left Ankle [m]" : Outport  Port=2
  Joint Angles Left [rad] : Outport  Port=3
  "Joint Velocities Left [rad/s] " : Outport  Port=4
  Joint Accelerations Left [rad/s^2] : Outport  Port=5
  tag scope: AnklePosL=global
  wires:
  extension definition1/1 -> Mux1/4, Ankle Mechanical Limits/1(dq [rad/s])
  A Pos Sensor/1 -> extension definition/1
  Ankle Mechanical Limits/1(tau [Nm]) -> Sum2/2
  A Vel Sensor/1 -> extension definition1/1
  Sum2/1 -> extensor definition/1
  "H Roll Vel Sensor "/1 -> Mux1/2, Hip Roll Mechanical Limits/1(dq [rad/s])
  K Vel Sensor/1 -> Mux1/3, Knee Mechanical Limits/1(dq [rad/s])
  Knee Mechanical Limits/1(tau [Nm]) -> Sum5/2
  Hip Roll Mechanical Limits/1(tau [Nm]) -> Sum1/2
  H Pitch Vel Sensor/1 -> Mux1/1, Hip Pitch Mechanical Limits/1(dq [rad/s])
  Hip Pitch Mechanical Limits/1(tau [Nm]) -> Sum4/2
  Sum4/1 -> H Pitch Actuator/1
  Sum1/1 -> H Roll Actuator/1
  Sum5/1 -> " K Actuator"/1
  extensor definition/1 -> A Actuator/1
  Mux1/1 -> "Joint Velocities Left [rad/s] "/1
  Mux2/1 -> Joint Accelerations Left [rad/s^2]/1
  H Pitch Acc Sensor/1 -> Mux2/1
  H Roll Acc Sensor/1 -> Mux2/2
  K Acc Sensor/1 -> Mux2/3
  A acc Sensor/1 -> extension definition2/1
  extension definition2/1 -> Mux2/4
  Demux/1 -> Sum4/1
  Demux/2 -> Sum1/1
  Demux/3 -> Sum5/1
  Demux/4 -> Sum2/1
  Sensor Left Ankle/1(Position [m]) -> " Position Left Ankle [m]"/1, Selector1/1, [AnklePosL]
  Rotation Sensor Knee/2(Rotation Matrix) -> Rotation Matrix Left Knee (world)/1
  Sensor Left Ankle/2(Velocity [m/s]) -> Terminator/1
  Torques [Nm]/1 -> Demux/1
  K Pos Sensor/1 -> Mux7/3, Knee Mechanical Limits/2(q [rad])  "qK"
  H Pitch Pos Sensor/1 -> Hip Pitch Mechanical Limits/2(q [rad]), Mux7/1  "qHP"
  H Roll Pos Sensor/1 -> Mux7/2, Hip Roll Mechanical Limits/2(q [rad])  "qHR"
  extension definition/1 -> Mux7/4, Ankle Mechanical Limits/2(q [rad])  "qA"
  Mux7/1 -> Joint Angles Left [rad]/1
  Rotation Sensor Knee/1(rotation [rad]) -> Terminator1/1
  Selector1/1 -> Compare To Constant1/1
  Compare To Constant1/1 -> Stop Simulation1/1
  connections:
  Left Ankle (LA) Pitch/RConn1 -- Sensor Left Ankle/LConn1 -- Foot/LConn1
  A Pos Sensor/LConn1 -- Left Ankle (LA) Pitch/RConn2
  A Vel Sensor/LConn1 -- Left Ankle (LA) Pitch/RConn3
  Left Ankle (LA) Pitch/LConn1 -- Shank/RConn1
  Left Hip (LH) Pitch (about X) and Roll (about Y) Joints/RConn1 -- LH Axis Inverse Rotation/LConn1
  Thigh/RConn1 -- Rotation Sensor Knee/LConn1 -- LK Axis Rotation/LConn1
  Shank/LConn1 -- Left Knee (LK) Pitch/RConn1
  Left Hip (LH) Pitch (about X) and Roll (about Y) Joints/LConn1 -- LH Axis Rotation/RConn1
  H Pitch Vel Sensor/LConn1 -- Left Hip (LH) Pitch (about X) and Roll (about Y) Joints/RConn3
  H Pitch Pos Sensor/LConn1 -- Left Hip (LH) Pitch (about X) and Roll (about Y) Joints/RConn2
  K Pos Sensor/LConn1 -- Left Knee (LK) Pitch/RConn2
  K Vel Sensor/LConn1 -- Left Knee (LK) Pitch/RConn3
  LH Axis Rotation/LConn1 -- Left Hip/RConn1
  Left Hip (LH) Pitch (about X) and Roll (about Y) Joints/RConn6 -- "H Roll Vel Sensor "/LConn1
  Left Hip (LH) Pitch (about X) and Roll (about Y) Joints/RConn5 -- H Roll Pos Sensor/LConn1
  Left Hip (LH) Pitch (about X) and Roll (about Y) Joints/RConn4 -- H Pitch Acc Sensor/LConn1
  Left Hip (LH) Pitch (about X) and Roll (about Y) Joints/RConn7 -- H Roll Acc Sensor/LConn1
  Left Knee (LK) Pitch/RConn4 -- K Acc Sensor/LConn1
  Left Ankle (LA) Pitch/RConn4 -- A acc Sensor/LConn1
  LK Axis Rotation/RConn1 -- Left Knee (LK) Pitch/LConn1
  Right Heel/RConn1 -- Foot/LConn3
  Foot/LConn2 -- Left Heel/RConn1
  Left Ball/RConn1 -- Foot/RConn1
  Right Ball/RConn1 -- Foot/RConn2
  Thigh/LConn1 -- LH Axis Inverse Rotation/RConn1
  " K Actuator"/RConn1 -- Left Knee (LK) Pitch/LConn2
  A Actuator/RConn1 -- Left Ankle (LA) Pitch/LConn2
  H Pitch Actuator/RConn1 -- Left Hip (LH) Pitch (about X) and Roll (about Y) Joints/LConn2
  H Roll Actuator/RConn1 -- Left Hip (LH) Pitch (about X) and Roll (about Y) Joints/LConn3

== system nmsRR/Body and Contact Model/LPF 13x0.01s1 ==
  in : Inport
  Demux2 : Demux  Outputs=13
  Mux2 : Mux  Inputs=13
  Transfer Fcn (with initial outputs)1 : simulink_extras/Additional Linear/Transfer Fcn (with initial outputs)  N=[1]  D="[0.01  1]"  Y0=init_sensor_body(1)  U0=init_sensor_body(1)
  Transfer Fcn (with initial outputs)10 : simulink_extras/Additional Linear/Transfer Fcn (with initial outputs)  N=[1]  D="[0.01  1]"  Y0=init_sensor_body(10)  U0=init_sensor_body(10)
  Transfer Fcn (with initial outputs)11 : simulink_extras/Additional Linear/Transfer Fcn (with initial outputs)  N=[1]  D="[0.01  1]"  Y0=init_sensor_body(11)  U0=init_sensor_body(11)
  Transfer Fcn (with initial outputs)12 : simulink_extras/Additional Linear/Transfer Fcn (with initial outputs)  N=[1]  D="[0.01  1]"  Y0=init_sensor_body(12)  U0=init_sensor_body(12)
  Transfer Fcn (with initial outputs)13 : simulink_extras/Additional Linear/Transfer Fcn (with initial outputs)  N=[1]  D="[0.01  1]"  Y0=init_sensor_body(13)  U0=init_sensor_body(13)
  Transfer Fcn (with initial outputs)2 : simulink_extras/Additional Linear/Transfer Fcn (with initial outputs)  N=[1]  D="[0.01  1]"  Y0=init_sensor_body(2)  U0=init_sensor_body(2)
  Transfer Fcn (with initial outputs)3 : simulink_extras/Additional Linear/Transfer Fcn (with initial outputs)  N=[1]  D="[0.01  1]"  Y0=init_sensor_body(3)  U0=init_sensor_body(3)
  Transfer Fcn (with initial outputs)4 : simulink_extras/Additional Linear/Transfer Fcn (with initial outputs)  N=[1]  D="[0.01  1]"  Y0=init_sensor_body(4)  U0=init_sensor_body(4)
  Transfer Fcn (with initial outputs)5 : simulink_extras/Additional Linear/Transfer Fcn (with initial outputs)  N=[1]  D="[0.01  1]"  Y0=init_sensor_body(5)  U0=init_sensor_body(5)
  Transfer Fcn (with initial outputs)6 : simulink_extras/Additional Linear/Transfer Fcn (with initial outputs)  N=[1]  D="[0.01  1]"  Y0=init_sensor_body(6)  U0=init_sensor_body(6)
  Transfer Fcn (with initial outputs)7 : simulink_extras/Additional Linear/Transfer Fcn (with initial outputs)  N=[1]  D="[0.01  1]"  Y0=init_sensor_body(7)  U0=init_sensor_body(7)
  Transfer Fcn (with initial outputs)8 : simulink_extras/Additional Linear/Transfer Fcn (with initial outputs)  N=[1]  D="[0.01  1]"  Y0=init_sensor_body(8)  U0=init_sensor_body(8)
  Transfer Fcn (with initial outputs)9 : simulink_extras/Additional Linear/Transfer Fcn (with initial outputs)  N=[1]  D="[0.01  1]"  Y0=init_sensor_body(9)  U0=init_sensor_body(9)
  Out : Outport
  wires:
  Mux2/1 -> Out/1
  Demux2/1 -> Transfer Fcn (with initial outputs)1/1
  Demux2/12 -> Transfer Fcn (with initial outputs)12/1
  Transfer Fcn (with initial outputs)6/1 -> Mux2/6
  Transfer Fcn (with initial outputs)3/1 -> Mux2/3
  Transfer Fcn (with initial outputs)10/1 -> Mux2/10
  Demux2/2 -> Transfer Fcn (with initial outputs)2/1
  Transfer Fcn (with initial outputs)12/1 -> Mux2/12
  Transfer Fcn (with initial outputs)7/1 -> Mux2/7
  Demux2/10 -> Transfer Fcn (with initial outputs)10/1
  Transfer Fcn (with initial outputs)9/1 -> Mux2/9
  Demux2/9 -> Transfer Fcn (with initial outputs)9/1
  in/1 -> Demux2/1
  Transfer Fcn (with initial outputs)4/1 -> Mux2/4
  Transfer Fcn (with initial outputs)8/1 -> Mux2/8
  Transfer Fcn (with initial outputs)5/1 -> Mux2/5
  Transfer Fcn (with initial outputs)11/1 -> Mux2/11
  Demux2/11 -> Transfer Fcn (with initial outputs)11/1
  Demux2/7 -> Transfer Fcn (with initial outputs)7/1
  Demux2/3 -> Transfer Fcn (with initial outputs)3/1
  Demux2/6 -> Transfer Fcn (with initial outputs)6/1
  Transfer Fcn (with initial outputs)1/1 -> Mux2/1
  Demux2/5 -> Transfer Fcn (with initial outputs)5/1
  Transfer Fcn (with initial outputs)2/1 -> Mux2/2
  Demux2/4 -> Transfer Fcn (with initial outputs)4/1
  Demux2/8 -> Transfer Fcn (with initial outputs)8/1
  Demux2/13 -> Transfer Fcn (with initial outputs)13/1
  Transfer Fcn (with initial outputs)13/1 -> Mux2/13

== system nmsRR/Body and Contact Model/LPF 13x0.01s2 ==
  in : Inport
  Demux2 : Demux  Outputs=12
  Mux2 : Mux  Inputs=12
  Transfer Fcn (with initial outputs)1 : simulink_extras/Additional Linear/Transfer Fcn (with initial outputs)  N=[1]  D="[0.01  1]"  Y0=init_sensor_world(1)  U0=init_sensor_world(1)
  Transfer Fcn (with initial outputs)10 : simulink_extras/Additional Linear/Transfer Fcn (with initial outputs)  N=[1]  D="[0.01  1]"  Y0=init_sensor_world(10)  U0=init_sensor_world(10)
  Transfer Fcn (with initial outputs)11 : simulink_extras/Additional Linear/Transfer Fcn (with initial outputs)  N=[1]  D="[0.01  1]"  Y0=init_sensor_world(11)  U0=init_sensor_world(11)
  Transfer Fcn (with initial outputs)12 : simulink_extras/Additional Linear/Transfer Fcn (with initial outputs)  N=[1]  D="[0.01  1]"  Y0=init_sensor_world(12)  U0=init_sensor_world(12)
  Transfer Fcn (with initial outputs)2 : simulink_extras/Additional Linear/Transfer Fcn (with initial outputs)  N=[1]  D="[0.01  1]"  Y0=init_sensor_world(2)  U0=init_sensor_world(2)
  Transfer Fcn (with initial outputs)3 : simulink_extras/Additional Linear/Transfer Fcn (with initial outputs)  N=[1]  D="[0.01  1]"  Y0=init_sensor_world(3)  U0=init_sensor_world(3)
  Transfer Fcn (with initial outputs)4 : simulink_extras/Additional Linear/Transfer Fcn (with initial outputs)  N=[1]  D="[0.01  1]"  Y0=init_sensor_world(4)  U0=init_sensor_world(4)
  Transfer Fcn (with initial outputs)5 : simulink_extras/Additional Linear/Transfer Fcn (with initial outputs)  N=[1]  D="[0.01  1]"  Y0=init_sensor_world(5)  U0=init_sensor_world(5)
  Transfer Fcn (with initial outputs)6 : simulink_extras/Additional Linear/Transfer Fcn (with initial outputs)  N=[1]  D="[0.01  1]"  Y0=init_sensor_world(6)  U0=init_sensor_world(6)
  Transfer Fcn (with initial outputs)7 : simulink_extras/Additional Linear/Transfer Fcn (with initial outputs)  N=[1]  D="[0.01  1]"  Y0=init_sensor_world(7)  U0=init_sensor_world(7)
  Transfer Fcn (with initial outputs)8 : simulink_extras/Additional Linear/Transfer Fcn (with initial outputs)  N=[1]  D="[0.01  1]"  Y0=init_sensor_world(8)  U0=init_sensor_world(8)
  Transfer Fcn (with initial outputs)9 : simulink_extras/Additional Linear/Transfer Fcn (with initial outputs)  N=[1]  D="[0.01  1]"  Y0=init_sensor_world(9)  U0=init_sensor_world(9)
  Out : Outport
  wires:
  Mux2/1 -> Out/1
  Demux2/1 -> Transfer Fcn (with initial outputs)1/1
  Demux2/12 -> Transfer Fcn (with initial outputs)12/1
  Transfer Fcn (with initial outputs)6/1 -> Mux2/6
  Transfer Fcn (with initial outputs)3/1 -> Mux2/3
  Transfer Fcn (with initial outputs)10/1 -> Mux2/10
  Demux2/2 -> Transfer Fcn (with initial outputs)2/1
  Transfer Fcn (with initial outputs)12/1 -> Mux2/12
  Transfer Fcn (with initial outputs)7/1 -> Mux2/7
  Demux2/10 -> Transfer Fcn (with initial outputs)10/1
  Transfer Fcn (with initial outputs)9/1 -> Mux2/9
  Demux2/9 -> Transfer Fcn (with initial outputs)9/1
  in/1 -> Demux2/1
  Transfer Fcn (with initial outputs)4/1 -> Mux2/4
  Transfer Fcn (with initial outputs)8/1 -> Mux2/8
  Transfer Fcn (with initial outputs)5/1 -> Mux2/5
  Transfer Fcn (with initial outputs)11/1 -> Mux2/11
  Demux2/11 -> Transfer Fcn (with initial outputs)11/1
  Demux2/7 -> Transfer Fcn (with initial outputs)7/1
  Demux2/3 -> Transfer Fcn (with initial outputs)3/1
  Demux2/6 -> Transfer Fcn (with initial outputs)6/1
  Transfer Fcn (with initial outputs)1/1 -> Mux2/1
  Demux2/5 -> Transfer Fcn (with initial outputs)5/1
  Transfer Fcn (with initial outputs)2/1 -> Mux2/2
  Demux2/4 -> Transfer Fcn (with initial outputs)4/1
  Demux2/8 -> Transfer Fcn (with initial outputs)8/1
